simulink model "solution"  (R2020a)
settings: Solver=VariableStepAuto  StartTime=0.0  StopTime=10.0  RelTol=1e-3
undefined symbols (not defined in the file): Desc100Hz, Desc25Hz, Desc5Hz
settings Model: Creator=Alexey  LastModifiedBy=Alexey

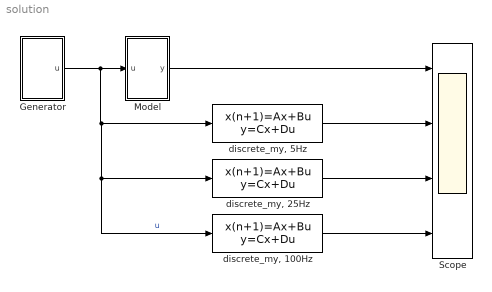
== system solution ==
  Generator : Subsystem
  Model : Subsystem
  Scope : Scope  NumInputPorts=4
  "discrete_my, 100Hz" : DiscreteStateSpace  A=Desc100Hz.Ad  B=Desc100Hz.Bd  C=Desc100Hz.Cd  D=Desc100Hz.Dd  SampleTime=1/100
  "discrete_my, 25Hz" : DiscreteStateSpace  A=Desc25Hz.Ad  B=Desc25Hz.Bd  C=Desc25Hz.Cd  D=Desc25Hz.Dd  SampleTime=1/25
  "discrete_my, 5Hz " : DiscreteStateSpace  A=Desc5Hz.Ad  B=Desc5Hz.Bd  C=Desc5Hz.Cd  D=Desc5Hz.Dd  SampleTime=1/5
  wires:
  Generator/1(u) -> "discrete_my, 100Hz"/1, "discrete_my, 25Hz"/1, "discrete_my, 5Hz "/1, Model/1(u)  "u"
  Model/1(y) -> Scope/1
  "discrete_my, 5Hz "/1 -> Scope/2
  "discrete_my, 25Hz"/1 -> Scope/3
  "discrete_my, 100Hz"/1 -> Scope/4

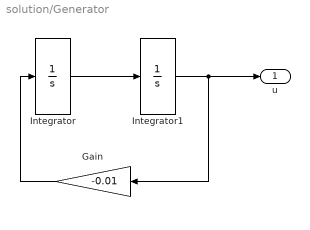
== system solution/Generator ==
  Gain : Gain  Gain=-0.01
  Integrator : Integrator  InitialCondition=-0.3*sin(1)
  Integrator1 : Integrator  InitialCondition=3*cos(1)
  u : Outport
  wires:
  Gain/1 -> Integrator/1
  Integrator1/1 -> u/1, Gain/1
  Integrator/1 -> Integrator1/1

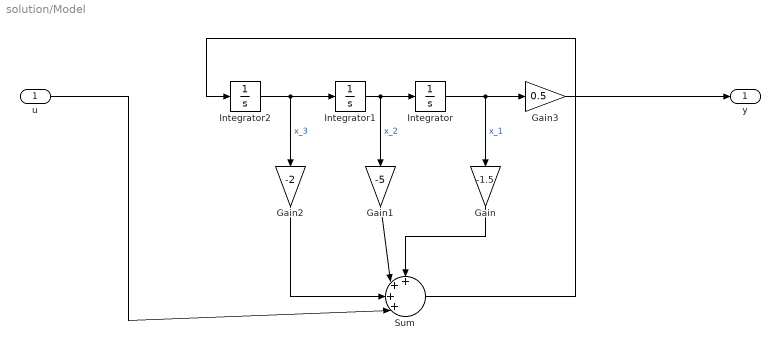
== system solution/Model ==
  u : Inport
  Gain : Gain  Gain=-1.5
  Gain1 : Gain  Gain=-5
  Gain2 : Gain  Gain=-2
  Gain3 : Gain  Gain=0.5
  Integrator : Integrator
  Integrator1 : Integrator
  Integrator2 : Integrator
  Sum : Sum  Inputs=++++|
  y : Outport
  wires:
  Sum/1 -> Integrator2/1
  Gain/1 -> Sum/1
  Integrator/1 -> Gain3/1, Gain/1  "x_1"
  Integrator2/1 -> Gain2/1, Integrator1/1  "x_3"
  Gain2/1 -> Sum/3
  Gain3/1 -> y/1
  u/1 -> Sum/4
  Integrator1/1 -> Integrator/1, Gain1/1  "x_2"
  Gain1/1 -> Sum/2
